simulink model "Diesel_Generator_Harness"  (R2025b)
settings: Solver=VariableStepAuto  StartTime=0.0  StopTime=15  RelTol=1e-3
PreLoadFcn:
  | GeneratorHarnessParam;
undefined symbols (not defined in the file): DiscIntNeverNeededParam, generator, machine, Ts
libraries: nesl_utility x16, ee_lib x14, fl_lib x7, eeGeneralControl x4, eeSmDC2C x1
settings Model: SimulationMode=accelerator  Creator=skota  LastModifiedBy=skota

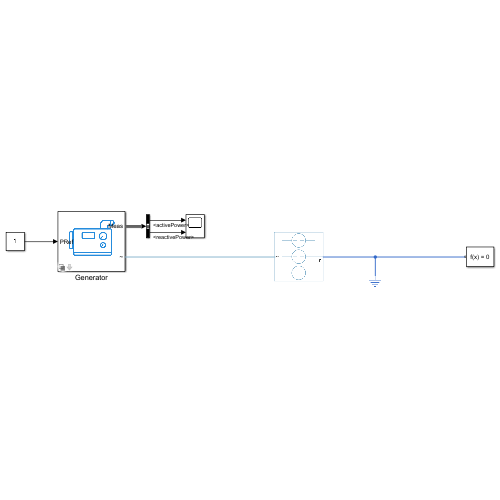
[thumbnail: Simulink's stored preview of the top-level diagram]
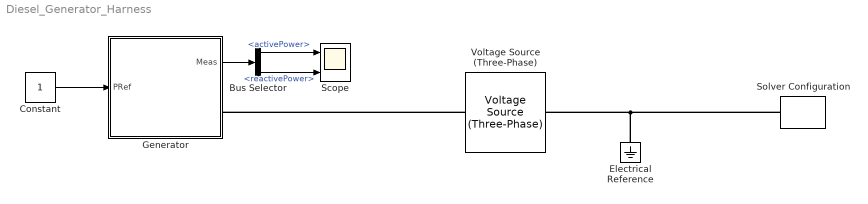
== system Diesel_Generator_Harness ==
  Bus Selector : BusSelector  OutputSignals=activePower,reactivePower
  Constant : Constant
  Electrical Reference : fl_lib/Electrical/Electrical Elements/Electrical Reference
  Generator : Subsystem  Variant=on  VariantControlMode=label  LabelModeActiveChoice=Detailed  mask(Generator){fidelity=Detailed, genRating=generator.rating, Vac=generator.Vac, frequency=generator.frequency, polePairs=generator.polePairs, pu_speed_reference=machine.speedReference, droop_percentage=machine.droop, pu_load_reference_setpoint=machine.loadReference, T_G=machine.timeConstandGovernor, T_CH=machine.timeConstantPrimeMover, base_torque=machine.baseTorque, pu_torque0=machine.initialTorque}
      mask prompts: fidelity "Modeling Option"; genRating "Generator Rating (kW)"; Vac "Rated AC side voltage (phase-phase RMS) (V)"; frequency "Rated electrical frequency at AC side (Hz)"; polePairs "Number of pole pairs"; pu_speed_reference "Speed reference, (pu)"; droop_percentage "Percentage droop, (%)"; pu_load_reference_setpoint "Load reference setpoint, (pu)"; T_G "Time constant of governor, (s)"; T_CH "Time constant of main inlet volumes and steam chest, (s)"; base_torque "Base torque, (N*m)"; pu_torque0 "Initial torque, (pu)"
      mask help:
      | This block models a Generator. The detailed variant models AVR, Exciter, Prime mover, and Governer. The simplified variant is based on load torque and a constant field circuit current. Select simplified mode for faster simulation using fixed efficiency and rated power.
      |
      | Provide load reference as input
      settings: CopyFcn=set_param(gcbh,'LinkStatus','none');
      mask Help: web('Generator.html')
      mask TypeOptions fidelity: Detailed | Simplified
      mask Callback fidelity:
      | detailedTabs = {'generatorDetailed','exciterParam','governerParam',};
      |     simplifiedTabs = {'generatorSimplified'};
      |     component.mask.fidelitySelection(detailedTabs,simplifiedTabs);
      |     component.mask.fidelitySelection;
      mask TypeOptions pu_speed_reference:
      | Detailed/Governor and
      | Prime Mover
      | /pu_speed_reference
      mask TypeOptions droop_percentage:
      | Detailed/Governor and
      | Prime Mover
      | /droop_percentage
      mask TypeOptions pu_load_reference_setpoint:
      | Detailed/Governor and
      | Prime Mover
      | /pu_load_reference_setpoint
      mask TypeOptions T_G:
      | Detailed/Governor and
      | Prime Mover
      | /T_G
      mask TypeOptions T_CH:
      | Detailed/Governor and
      | Prime Mover
      | /T_CH
      mask TypeOptions base_torque:
      | Detailed/Governor and
      | Prime Mover
      | /base_torque
      mask TypeOptions pu_torque0:
      | Detailed/Governor and
      | Prime Mover
      | /pu_torque0
      mask DialogControl generalDetailed Prompt: General
      mask DialogControl editMachine Prompt: Edit machine parameters
      mask DialogControl editMachine Callback:
      | blockFidelity = get_param(gcb,'fidelity');
      |     blockPath = [gcb,'/',blockFidelity,'/','Machine'];
      |     component.mask.openBlock(blockPath);
      mask DialogControl editInertia Prompt: Edit inertia parameters
      mask DialogControl editInertia Callback:
      | blockPath = [gcb,'/','Detailed','/','Inertia'];
      |     component.mask.openBlock(blockPath);
      mask DialogControl exciterParam Prompt: Exciter
      mask DialogControl fieldParam Prompt: Edit field circuit parameters
      mask DialogControl fieldParam Callback:
      | blockPath = [gcb,'/','Detailed','/','AVR and Exciter','/','Exciter'];
      |     component.mask.openBlock(blockPath);
      mask DialogControl avrParam Prompt: Edit AVR parameters
      mask DialogControl avrParam Callback:
      | blockPath = [gcb,'/','Detailed','/','AVR and Exciter','/','AVR'];
      |     component.mask.openBlock(blockPath);
      mask DialogControl governerParam Prompt: Governer and Prime Mover
  Scope : Scope  NumInputPorts=2
      settings: ActiveDisplayYMinimum=-1.6422066833599676  ActiveDisplayYMaximum=1.1874659177964262
  Solver Configuration : nesl_utility/Solver Configuration  PhysicalDomain=network_engine_domain  SubClassName=solver  LeftPortType=input  RightPortType=generic  Tones=[]  Harmonics=[]  SimulateNoise=off  Profile=off  UseLocalSampling=off  EnableSwitchedLinearOptims=on  FrequencyDomain=off  UseCCode=off  RelTol=0.001  AbsTol=0.001  MinStep=1e-09  ToWorkspace=off  RevertToSquareIcSolve=off  NumHomotopyIterations=100  PhasorMode=off  PhasorModeNumHarmonics=1  ConsistencySolver=NEWTON_XTOL_AFTER_FTOL  IndexReductionMethod=DerivativeReplacement  DoDC=off  ResidualTolerance=1e-09  ConsistencyTolSource=GLOBAL  ConsistencyAbsTol=0.001  ConsistencyRelTol=0.001  ConsistencyTolFactor=0.001  UseLocalSolver=on  LocalSolverChoice=NE_BACKWARD_EULER_ADVANCER  ResolveIndetEquations=on  FunctionEvalNumThread=1  LocalSolverSampleTime=5e-5  DoFixedCost=off  MaxNonlinIter=3  MaxModeIter=2  ComputeImpulses=off  ImpulseIterations=2  LinearAlgebra=auto  LinearAlgebraNumThread=0  EquationFormulation=NE_TIME_EF  DelaysMemoryBudget=1024  AutomaticFiltering=on  FilteringTimeConstant=0.001  PartitionStorageMethod=AS_NEEDED  PartitionMemoryBudget=1024  PartitionMethod=ROBUST  MultibodyUseLocalSolver=off  MultibodyLocalSolverChoice=ODE1  MultibodyLocalSolverSampleTime=0.001
  Voltage Source (Three-Phase) : ee_lib/Sources/Voltage Source (Three-Phase)  vline_rms=480 V  shift=0 deg  freq=60 Hz  impedance_option=1  SShortCircuit=100e6 A*V  XR=20  R=0.01 Ohm  L=3.97e-4 H  harmonic_option=0  harmonic_orders=[5, 7, 11, 13]  harmonic_ratios=[.1, .1, .1, .1]  G_parasitic=0 1/Ohm  I_specify=off  I_priority=None  I=[0, 0, 0] A  I_nominal_specify=off  I_nominal_value=1  I_nominal_unit=A
  wires:
  Bus Selector/1 -> Scope/1  "<activePower>"
  Bus Selector/2 -> Scope/2  "<reactivePower>"
  Constant/1 -> Generator/1(PRef)
  Generator/1(Meas) -> Bus Selector/1
  connections:
  Electrical Reference/LConn1 -- Solver Configuration/RConn1 -- Voltage Source (Three-Phase)/LConn1
  Voltage Source (Three-Phase)/RConn1 -- Generator/RConn1

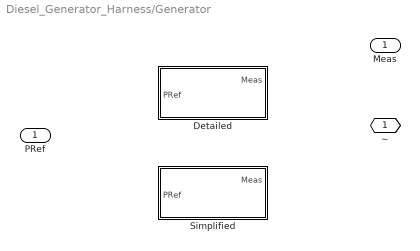
== system Diesel_Generator_Harness/Generator ==
  PRef : Inport
  Detailed : Subsystem  VariantControl=Detailed
  Simplified : Subsystem  VariantControl=Simplified
  ~ : PMIOPort  Side=Right
  Meas : Outport

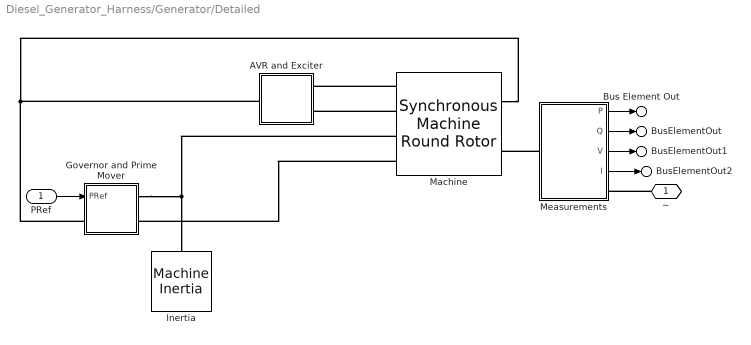
== system Diesel_Generator_Harness/Generator/Detailed ==
  PRef : Inport
  AVR and Exciter : Subsystem
  "Governor and Prime Mover " : Subsystem  mask(Governor and Prime Mover){pu_speed_reference=pu_speed_reference, droop_percentage=droop_percentage, pu_load_reference_setpoint=pu_load_reference_setpoint, T_G=T_G, T_CH=T_CH, base_torque=base_torque, pu_torque0=pu_torque0}
      mask prompts: pu_speed_reference "Speed reference, (pu)"; droop_percentage "Percentage droop, (%)"; pu_load_reference_setpoint "Load reference setpoint, (pu)"; T_G "Time constant of governor, (s)"; T_CH "Time constant of main inlet volumes and steam chest, (s)"; base_torque "Base torque, (N*m)"; pu_torque0 "Initial torque, (pu)"
      mask help:
      | Implements a synchronous machine governor and prime mover. The prime mover is a non-reheat steam turbine.
      |
      | The input to the block is a per-unit synchronous machine measurement vector.
      |
      | R and C are mechanical rotational ports.
  Inertia : ee_lib/Electromechanical/Mechanical/Machine Inertia  SRated=genRating*1000 V*A  FRated=frequency Hz  nPolePairs=polePairs  inertia_option=2  J=0.5754*200 kg*m^2  H=3.525*2 s*W/V/A  damper_option=2  D=39.0509 N*m/(rad/s)  pu_D=0.01  initialization_option=2  fMechanical0=60 Hz  fElectrical0=frequency Hz
      settings: InternalSimscapePortConfiguration="{\"Bottom\":[],\"Left\":[{\"id\":\"R\",\"label\":\"R\",\"type\":\"foundation.mechanical.rotational.rotational\"}],\"Right\":[],\"Top\":[]}"
  Machine : ee_lib/Electromechanical/Synchronous/Synchronous Machine Round Rotor  port_option=ee.enum.threePhasePort.composite  SRated=genRating*1000 A*V  VRated=Vac V  FRated=frequency Hz  nPolePairs=polePairs  param_option=ee.enum.sm.parameterization.standard  fieldCircuitParameterization_option=ee.enum.sm.fieldparameterization.current  baseEfd=92.95 V  baseIfd=machine.fieldCurrent A  zero_sequence=ee.enum.park.zerosequence.exclude  axes_param=ee.enum.rotorangle.daxis  Ladu=1.66  Laqu=1.61  L0=0.15  Ll=0.05  Ra=machine.Ra/2  Lfd=0.165  Rfd=0.0006  L1d=0.1713  R1d=0.0284  L1q=0.7252  R1q=0.00619  L2q=0.125  R2q=0.02368  Xl=machine.Xl  Xd=machine.Xd  Xq=machine.Xq  X0=0.06  Xdd=machine.XdTransient  Xqd=machine.XqTransient  Xddd=machine.XdSubTransient  Xqdd=machine.XqSubTransient  d_option=ee.enum.circuit.open  Td0d=machine.tauDAxisTransient s  Tdd=0.03 s  Td0dd=machine.tauDAxisSubTransient s  Tddd=0.008 s  q_option=ee.enum.circuit.open  Tq0d=machine.tauQAxisTransient s  Tqd=0.03 s  Tq0dd=machine.tauQAxisSubTransient s  Tqdd=0.008 s  saturation_option=ee.enum.saturation.exclude  saturation_ifd=[0, .48, .76, 1.38, 1.79]  saturation_Vag=[0, .8, 1.08, 1.31, 1.4]  initialization_option=ee.enum.sm.initialization.steadystate  source_type=ee.enum.sm.load_flow_source_type.Swing  Vmag0=machine.voltage V  Vang0=0 deg  Pt0=0 A*V  Qt0=0 A*V  minimum_pu=0.95  phase_search_range=[-inf, inf] deg  gmin=1e-6 S  connection_option=ee.enum.Connection.wye  num_q_dampers=2  rotor_offset=-pi / 2 rad  pu_psid_specify=off  pu_psid_priority=None  pu_psid=0  pu_psid_nominal_specify=off  pu_psid_nominal_value=1  pu_psid_nominal_unit=1  pu_psiq_specify=off  pu_psiq_priority=None  pu_psiq=0  pu_psiq_nominal_specify=off  pu_psiq_nominal_value=1  pu_psiq_nominal_unit=1  pu_psifd_specify=off  pu_psifd_priority=None  pu_psifd=0  pu_psifd_nominal_specify=off  pu_psifd_nominal_value=1  pu_psifd_nominal_unit=1  pu_psi1d_specify=off  pu_psi1d_priority=None  pu_psi1d=0  pu_psi1d_nominal_specify=off  pu_psi1d_nominal_value=1  pu_psi1d_nominal_unit=1  pu_psi1q_specify=off  pu_psi1q_priority=None  pu_psi1q=0  pu_psi1q_nominal_specify=off  pu_psi1q_nominal_value=1  pu_psi1q_nominal_unit=1  pu_psi2q_specify=off  pu_psi2q_priority=None  pu_psi2q=0  pu_psi2q_nominal_specify=off  pu_psi2q_nominal_value=1  pu_psi2q_nominal_unit=1  angular_position_diff_specify=off  angular_position_diff_priority=None  angular_position_diff=180 deg  angular_position_diff_nominal_specify=off  angular_position_diff_nominal_value=1  angular_position_diff_nominal_unit=deg  Tmeas=298.15 K  alpha=3.93e-3 1/K  stator_thermal_mass=100 J/K  rotor_thermal_mass=200 J/K  temperatureA_specify=off  temperatureA_priority=High  temperatureA=25 degC  temperatureA_nominal_specify=off  temperatureA_nominal_value=1  temperatureA_nominal_unit=degC  temperatureB_specify=off  temperatureB_priority=High  temperatureB=25 degC  temperatureB_nominal_specify=off  temperatureB_nominal_value=1  temperatureB_nominal_unit=degC  temperatureC_specify=off  temperatureC_priority=High  temperatureC=25 degC  temperatureC_nominal_specify=off  temperatureC_nominal_value=1  temperatureC_nominal_unit=degC  temperatureR_specify=off  temperatureR_priority=High  temperatureR=25 degC  temperatureR_nominal_specify=off  temperatureR_nominal_value=1  temperatureR_nominal_unit=degC
      settings: InternalSimscapePortConfiguration="{\"Bottom\":[],\"Left\":[{\"id\":\"fd_p\",\"label\":\"fd+\",\"type\":\"foundation.electrical.electrical\"},{\"id\":\"fd_n\",\"label\":\"fd-\",\"type\":\"foundation.electrical.electrical\"},{\"id\":\"R\",\"label\":\"R\",\"type\":\"foundation.mechanical.rotational.rotational\"},{\"id\":\"C\",\"label\":\"C\",\"type\":\"foundation.mechanical.rotational.rotational\"}],\"Right\":[{\"id\":\"pu_output\",\"label\":\"pu\",\"type\":\"output\"},{\"id\":\"N\",\"label\":\"~\",\"type\":\"foundation.electrical.three_phase\"}],\"Top\":[]}"
  Measurements : Subsystem
  ~ : PMIOPort  Side=Right
  Bus Element Out : Outport  PortName=Meas  Element=activePower
  BusElementOut : Outport  PortName=Meas  Element=reactivePower
  BusElementOut1 : Outport  PortName=Meas  Element=voltage
  BusElementOut2 : Outport  PortName=Meas  Element=current
  wires:
  Measurements/4(I) -> BusElementOut2/1
  Measurements/3(V) -> BusElementOut1/1
  Measurements/1(P) -> Bus Element Out/1
  Measurements/2(Q) -> BusElementOut/1
  PRef/1 -> "Governor and Prime Mover "/1(PRef)
  connections:
  ~/RConn1 -- Measurements/RConn1
  Measurements/LConn1 -- Machine/RConn2
  Machine/LConn1 -- AVR and Exciter/RConn1
  Machine/LConn4 -- "Governor and Prime Mover "/RConn2
  "Governor and Prime Mover "/RConn1 -- Machine/LConn3 -- Inertia/LConn1
  "Governor and Prime Mover "/LConn1 -- Machine/RConn1 -- AVR and Exciter/LConn1
  Machine/LConn2 -- AVR and Exciter/RConn2

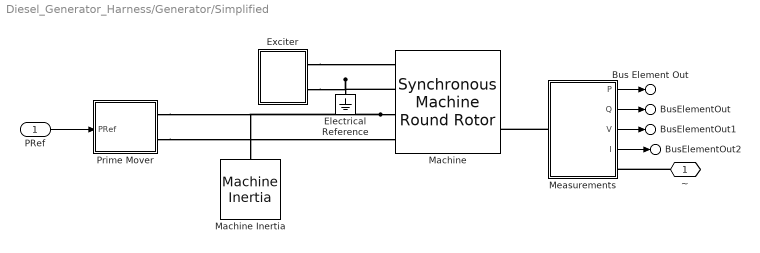
== system Diesel_Generator_Harness/Generator/Simplified ==
  PRef : Inport
  Electrical Reference : fl_lib/Electrical/Electrical Elements/Electrical Reference
  Exciter : Subsystem
  Machine : ee_lib/Electromechanical/Synchronous/Synchronous Machine Round Rotor  port_option=ee.enum.threePhasePort.composite  SRated=genRating kW  VRated=Vac V  FRated=frequency Hz  nPolePairs=polePairs  param_option=ee.enum.sm.parameterization.standard  fieldCircuitParameterization_option=ee.enum.sm.fieldparameterization.voltage  baseEfd=100 V  baseIfd=1300 A  zero_sequence=ee.enum.park.zerosequence.exclude  axes_param=ee.enum.rotorangle.daxis  Ladu=1.66  Laqu=1.61  L0=0.15  Ll=0.05  Ra=0.03/5  Lfd=0.165  Rfd=0.0006  L1d=0.1713  R1d=0.0284  L1q=0.7252  R1q=0.00619  L2q=0.125  R2q=0.02368  Xl=0.05/5  Xd=1.72/5  Xq=0.79/5  X0=0.06  Xdd=0.13/5  Xqd=0.17/3  Xddd=0.09/5  Xqdd=0.12/5  d_option=ee.enum.circuit.short  Td0d=0.75 s  Tdd=0.03 s  Td0dd=0.03 s  Tddd=0.008 s  q_option=ee.enum.circuit.open  Tq0d=0.6 s  Tqd=0.03 s  Tq0dd=0.02 s  Tqdd=0.008 s  saturation_option=ee.enum.saturation.exclude  saturation_ifd=[0, .48, .76, 1.38, 1.79]  saturation_Vag=[0, .8, 1.08, 1.31, 1.4]  initialization_option=ee.enum.sm.initialization.steadystate  source_type=ee.enum.sm.load_flow_source_type.Swing  Vmag0=6600 V  Vang0=0 deg  Pt0=0 A*V  Qt0=0 A*V  minimum_pu=0.95  phase_search_range=[-inf, inf] deg  gmin=1e-4 S  connection_option=ee.enum.Connection.wye  num_q_dampers=2  rotor_offset=-pi / 2 rad  pu_psid_specify=off  pu_psid_priority=None  pu_psid=0  pu_psid_nominal_specify=off  pu_psid_nominal_value=1  pu_psid_nominal_unit=1  pu_psiq_specify=off  pu_psiq_priority=None  pu_psiq=0  pu_psiq_nominal_specify=off  pu_psiq_nominal_value=1  pu_psiq_nominal_unit=1  pu_psifd_specify=off  pu_psifd_priority=None  pu_psifd=0  pu_psifd_nominal_specify=off  pu_psifd_nominal_value=1  pu_psifd_nominal_unit=1  pu_psi1d_specify=off  pu_psi1d_priority=None  pu_psi1d=0  pu_psi1d_nominal_specify=off  pu_psi1d_nominal_value=1  pu_psi1d_nominal_unit=1  pu_psi1q_specify=off  pu_psi1q_priority=None  pu_psi1q=0  pu_psi1q_nominal_specify=off  pu_psi1q_nominal_value=1  pu_psi1q_nominal_unit=1  pu_psi2q_specify=off  pu_psi2q_priority=None  pu_psi2q=0  pu_psi2q_nominal_specify=off  pu_psi2q_nominal_value=1  pu_psi2q_nominal_unit=1  angular_position_diff_specify=off  angular_position_diff_priority=None  angular_position_diff=180 deg  angular_position_diff_nominal_specify=off  angular_position_diff_nominal_value=1  angular_position_diff_nominal_unit=deg  Tmeas=298.15 K  alpha=3.93e-3 1/K  stator_thermal_mass=100 J/K  rotor_thermal_mass=200 J/K  temperatureA_specify=off  temperatureA_priority=High  temperatureA=25 degC  temperatureA_nominal_specify=off  temperatureA_nominal_value=1  temperatureA_nominal_unit=degC  temperatureB_specify=off  temperatureB_priority=High  temperatureB=25 degC  temperatureB_nominal_specify=off  temperatureB_nominal_value=1  temperatureB_nominal_unit=degC  temperatureC_specify=off  temperatureC_priority=High  temperatureC=25 degC  temperatureC_nominal_specify=off  temperatureC_nominal_value=1  temperatureC_nominal_unit=degC  temperatureR_specify=off  temperatureR_priority=High  temperatureR=25 degC  temperatureR_nominal_specify=off  temperatureR_nominal_value=1  temperatureR_nominal_unit=degC
      settings: InternalSimscapePortConfiguration="{\"Bottom\":[],\"Left\":[{\"id\":\"fd_p\",\"label\":\"fd+\",\"type\":\"foundation.electrical.electrical\"},{\"id\":\"fd_n\",\"label\":\"fd-\",\"type\":\"foundation.electrical.electrical\"},{\"id\":\"R\",\"label\":\"R\",\"type\":\"foundation.mechanical.rotational.rotational\"},{\"id\":\"C\",\"label\":\"C\",\"type\":\"foundation.mechanical.rotational.rotational\"}],\"Right\":[{\"id\":\"pu_output\",\"label\":\"pu\",\"type\":\"output\"},{\"id\":\"N\",\"label\":\"~\",\"type\":\"foundation.electrical.three_phase\"}],\"Top\":[]}"
  Machine Inertia : ee_lib/Electromechanical/Mechanical/Machine Inertia  SRated=genRating*1000 V*A  FRated=frequency Hz  nPolePairs=polePairs  inertia_option=1  J=0.5754 kg*m^2  H=3.525 s*W/V/A  damper_option=2  D=39.0509 N*m/(rad/s)  pu_D=0.01  initialization_option=2  fMechanical0=60 Hz  fElectrical0=60 Hz
      settings: InternalSimscapePortConfiguration="{\"Bottom\":[],\"Left\":[{\"id\":\"R\",\"label\":\"R\",\"type\":\"foundation.mechanical.rotational.rotational\"}],\"Right\":[],\"Top\":[]}"
  Measurements : Subsystem
  Prime Mover : Subsystem
  ~ : PMIOPort  Side=Right
  Bus Element Out : Outport  PortName=Meas  Element=activePower
  BusElementOut : Outport  PortName=Meas  Element=reactivePower
  BusElementOut1 : Outport  PortName=Meas  Element=voltage
  BusElementOut2 : Outport  PortName=Meas  Element=current
  wires:
  Measurements/2(Q) -> BusElementOut/1
  Measurements/1(P) -> Bus Element Out/1
  Measurements/3(V) -> BusElementOut1/1
  Measurements/4(I) -> BusElementOut2/1
  PRef/1 -> Prime Mover/1(PRef)
  connections:
  Measurements/LConn1 -- Machine/RConn2
  ~/RConn1 -- Measurements/RConn1
  Prime Mover/RConn2 -- Machine/LConn4
  Exciter/RConn1 -- Machine/LConn1
  Machine/LConn3 -- Prime Mover/RConn1 -- Machine Inertia/LConn1
  Electrical Reference/LConn1 -- Machine/LConn2 -- Exciter/RConn2

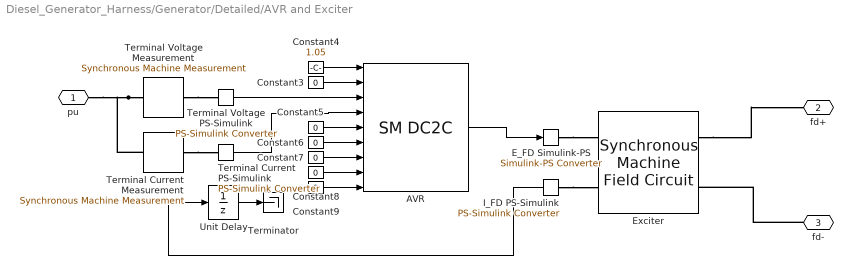
== system Diesel_Generator_Harness/Generator/Detailed/AVR and Exciter ==
  AVR : eeSmDC2C/SM DC2C  E_FD0=1.01  Ts=Ts  R_C=0  X_C=0  T_R=0  K_A=300  T_A=0.06  T_B=0  T_C=0  K_F=0.058  T_F=0.62  V_Rmax=4.5  V_Rmin=-4.5  oelInputLocation=Unused  uelInputLocation=Unused  sclInputLocation=Unused  K_E=1  T_E=1.33  E_FDmin=-99  E_1=3.05  S_E_E1=0.279  E_2=2.29  S_E_E2=0.117
  Constant{3,5..9} (6 alike) : Constant  Value=0
  Constant4 : Constant  Value=1.05
  "E_FD Simulink-PS " : nesl_utility/Simulink-PS Converter  PhysicalDomain=network_engine_domain  SubClassName=ps_input  LeftPortType=input  RightPortType=output  PseudoPeriodic=off  Frequencies=[]  NoiseDistribution=none  NoiseParameters=[]  Unit=1  AffineConversion=off  FilteringAndDerivatives=provide  SimscapeFilterOrder=1  InputFilterTimeConstant=.001  UdotUserProvided=0
  Exciter : ee_lib/Electromechanical/Synchronous/Synchronous Machine Field Circuit  unit_option=ee.enum.unit.pu  SRated=machine.ratedPower V*A  FRated=machine.frequency Hz  fieldCircuitParameterization_option=ee.enum.sm.fieldparameterization.current  baseEfd=200 V  baseIfd=machine.fieldCurrent A  parameterization_option=2  Ladu=1.66  Rfd=0.0006  Xl=machine.Xl  Xd=machine.Xd  Xdd=machine.XdTransient  Xddd=machine.XdSubTransient  d_option=ee.enum.circuit.open  Td0d=machine.tauDAxisTransient s  Tdd=0.03 s  Td0dd=machine.tauDAxisSubTransient s  Tddd=0.008 s
      settings: InternalSimscapePortConfiguration="{\"Bottom\":[],\"Left\":[{\"id\":\"Efd_pu\",\"label\":\"Efd_pu\",\"type\":\"input\"},{\"id\":\"Ifd_pu\",\"label\":\"Ifd_pu\",\"type\":\"output\"}],\"Right\":[{\"id\":\"fd_p\",\"label\":\"fd+\",\"type\":\"foundation.electrical.electrical\"},{\"id\":\"fd_n\",\"label\":\"fd-\",\"type\":\"foundation.electrical.electrical\"}],\"Top\":[]}"
  I_FD PS-Simulink : nesl_utility/PS-Simulink Converter  PhysicalDomain=network_engine_domain  SubClassName=ps_output  LeftPortType=input  RightPortType=output  PseudoPeriodic=off  Frequencies=[]  VectorFormat=1-D array  Unit=1  AffineConversion=off
  Terminal Current Measurement : ee_lib/Electromechanical/Synchronous/Synchronous Machine Measurement  output_idx=15
      settings: InternalSimscapePortConfiguration="{\"Bottom\":[],\"Left\":[{\"id\":\"pu_input\",\"label\":\"pu\",\"type\":\"input\"}],\"Right\":[{\"id\":\"pu_output\",\"label\":\"o\",\"type\":\"output\"}],\"Top\":[]}"
  Terminal Current PS-Simulink : nesl_utility/PS-Simulink Converter  PhysicalDomain=network_engine_domain  SubClassName=ps_output  LeftPortType=input  RightPortType=output  PseudoPeriodic=off  Frequencies=[]  VectorFormat=1-D array  Unit=1  AffineConversion=off
  Terminal Voltage Measurement : ee_lib/Electromechanical/Synchronous/Synchronous Machine Measurement  output_idx=14
      settings: InternalSimscapePortConfiguration="{\"Bottom\":[],\"Left\":[{\"id\":\"pu_input\",\"label\":\"pu\",\"type\":\"input\"}],\"Right\":[{\"id\":\"pu_output\",\"label\":\"o\",\"type\":\"output\"}],\"Top\":[]}"
  Terminal Voltage PS-Simulink : nesl_utility/PS-Simulink Converter  PhysicalDomain=network_engine_domain  SubClassName=ps_output  LeftPortType=input  RightPortType=output  PseudoPeriodic=off  Frequencies=[]  VectorFormat=1-D array  Unit=1  AffineConversion=off
  Terminator : Terminator
  Unit Delay : UnitDelay  InitialCondition=1.32943  SampleTime=-1
  pu : PMIOPort  Side=Left
  fd+ : PMIOPort  Port=2  Side=Right
  fd- : PMIOPort  Port=3  Side=Right
  wires:
  Unit Delay/1 -> Terminator/1
  I_FD PS-Simulink/1 -> Unit Delay/1
  Terminal Voltage PS-Simulink/1 -> AVR/3
  Constant3/1 -> AVR/2
  Constant4/1 -> AVR/1
  Constant5/1 -> AVR/5
  Constant6/1 -> AVR/6
  Constant7/1 -> AVR/7
  Constant8/1 -> AVR/8
  Constant9/1 -> AVR/9
  AVR/1 -> "E_FD Simulink-PS "/1
  Terminal Current PS-Simulink/1 -> AVR/4
  connections:
  "E_FD Simulink-PS "/RConn1 -- Exciter/LConn1
  I_FD PS-Simulink/LConn1 -- Exciter/LConn2
  fd-/RConn1 -- Exciter/RConn2
  Exciter/RConn1 -- fd+/RConn1
  Terminal Voltage Measurement/LConn1 -- Terminal Current Measurement/LConn1 -- pu/RConn1
  Terminal Voltage Measurement/RConn1 -- Terminal Voltage PS-Simulink/LConn1
  Terminal Current Measurement/RConn1 -- Terminal Current PS-Simulink/LConn1

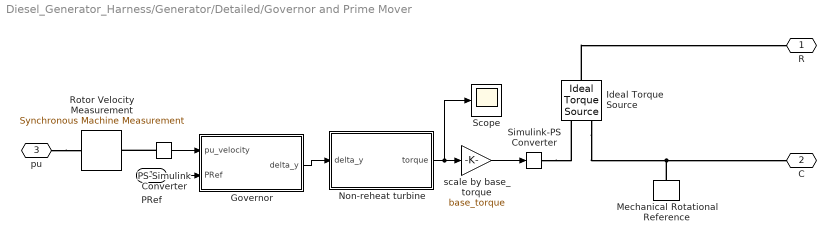
== system Diesel_Generator_Harness/Generator/Detailed/Governor and Prime Mover  ==
  PRef : Inport
  Governor : Subsystem
  Ideal Torque Source : fl_lib/Mechanical/Mechanical Sources/Ideal Torque Source
  Mechanical Rotational Reference : fl_lib/Mechanical/Rotational Elements/Mechanical Rotational Reference
  Non-reheat turbine : Subsystem
  PS-Simulink Converter : nesl_utility/PS-Simulink Converter  PhysicalDomain=network_engine_domain  SubClassName=ps_output  LeftPortType=input  RightPortType=output  PseudoPeriodic=off  Frequencies=[]  VectorFormat=1-D array  Unit=1  AffineConversion=off
  Rotor Velocity Measurement : ee_lib/Electromechanical/Synchronous/Synchronous Machine Measurement  output_idx=4
      settings: InternalSimscapePortConfiguration="{\"Bottom\":[],\"Left\":[{\"id\":\"pu_input\",\"label\":\"pu\",\"type\":\"input\"}],\"Right\":[{\"id\":\"pu_output\",\"label\":\"o\",\"type\":\"output\"}],\"Top\":[]}"
  Scope : Scope
  Simulink-PS Converter : nesl_utility/Simulink-PS Converter  PhysicalDomain=network_engine_domain  SubClassName=ps_input  LeftPortType=input  RightPortType=output  PseudoPeriodic=off  Frequencies=[]  NoiseDistribution=none  NoiseParameters=[]  Unit=1  AffineConversion=off  FilteringAndDerivatives=zero  SimscapeFilterOrder=1  InputFilterTimeConstant=0.001  UdotUserProvided=1
  scale by base_torque : Gain  Gain=base_torque
  R : PMIOPort  Side=Right
  C : PMIOPort  Port=2  Side=Right
  pu : PMIOPort  Port=3  Side=Left
  wires:
  PRef/1 -> Governor/2(PRef)
  scale by base_torque/1 -> Simulink-PS Converter/1
  Non-reheat turbine/1(torque) -> scale by base_torque/1, Scope/1
  Governor/1(delta_y) -> Non-reheat turbine/1(delta_y)
  PS-Simulink Converter/1 -> Governor/1(pu_velocity)
  connections:
  Simulink-PS Converter/RConn1 -- Ideal Torque Source/RConn1
  PS-Simulink Converter/LConn1 -- Rotor Velocity Measurement/RConn1
  pu/RConn1 -- Rotor Velocity Measurement/LConn1
  Ideal Torque Source/LConn1 -- R/RConn1
  Mechanical Rotational Reference/LConn1 -- Ideal Torque Source/RConn2 -- C/RConn1

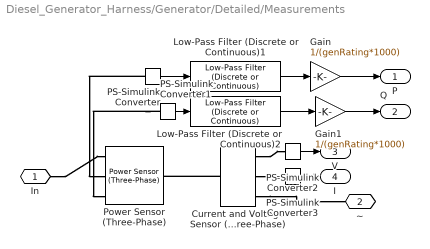
== system Diesel_Generator_Harness/Generator/Detailed/Measurements ==
  Current and Voltage Sensor (Three-Phase) : ee_lib/Sensors & Transducers/Current and Voltage Sensor (Three-Phase)  vMeasurementType=ee.enum.vmeasurement.ll  outputUnit=ee.enum.unit.pu  SRated=genRating*1000 A*V  VRated=Vac V  I_specify=off  I_priority=None  I=[0, 0, 0] A  I_nominal_specify=off  I_nominal_value=1  I_nominal_unit=A  V_specify=off  V_priority=None  V=[0, 0, 0] V  V_nominal_specify=off  V_nominal_value=1  V_nominal_unit=V
      settings: InternalSimscapePortConfiguration="{\"Bottom\":[],\"Left\":[{\"id\":\"N1\",\"label\":\"~1\",\"type\":\"foundation.electrical.three_phase\"}],\"Right\":[{\"id\":\"V_output\",\"label\":\"V\",\"type\":\"output\"},{\"id\":\"I_output\",\"label\":\"I\",\"type\":\"output\"},{\"id\":\"N2\",\"label\":\"~2\",\"type\":\"foundation.electrical.three_phase\"}],\"Top\":[]}"
  Gain : Gain  Gain=1/(genRating*1000)
  Gain1 : Gain  Gain=1/(genRating*1000)
  Low-Pass Filter (Discrete or Continuous)1 : eeGeneralControl/Low-Pass Filter (Discrete or Continuous)  K=1  T=0.1  B=inf  A=-inf  init_option=Inherited from block input  x0=0  Ts=-1
  Low-Pass Filter (Discrete or Continuous)2 : eeGeneralControl/Low-Pass Filter (Discrete or Continuous)  K=1  T=0.1  B=inf  A=-inf  init_option=Inherited from block input  x0=0  Ts=-1
  PS-Simulink Converter{,1..3} (4 alike) : nesl_utility/PS-Simulink Converter  PhysicalDomain=network_engine_domain  SubClassName=ps_output  LeftPortType=input  RightPortType=output  PseudoPeriodic=off  Frequencies=[]  VectorFormat=inherit  Unit=inherit  AffineConversion=off
  Power Sensor (Three-Phase) : ee_lib/Sensors & Transducers/Power Sensor (Three-Phase)  load_type=ee.enum.passive.type_balanced.balanced  f0=60 Hz
      settings: InternalSimscapePortConfiguration="{\"Bottom\":[],\"Left\":[{\"id\":\"N1\",\"label\":\"~1\",\"type\":\"foundation.electrical.three_phase\"}],\"Right\":[{\"id\":\"N2\",\"label\":\"~2\",\"type\":\"foundation.electrical.three_phase\"}],\"Top\":[{\"id\":\"Pm\",\"label\":\"P\",\"type\":\"output\"},{\"id\":\"Qm\",\"label\":\"Q\",\"type\":\"output\"}]}"
  In : PMIOPort  Side=Left
  ~ : PMIOPort  Port=2  Side=Right
  P : Outport
  Q : Outport  Port=2
  V : Outport  Port=3
  I : Outport  Port=4
  wires:
  Gain1/1 -> Q/1
  Gain/1 -> P/1
  PS-Simulink Converter3/1 -> I/1
  PS-Simulink Converter2/1 -> V/1
  Low-Pass Filter (Discrete or Continuous)2/1 -> Gain1/1
  Low-Pass Filter (Discrete or Continuous)1/1 -> Gain/1
  PS-Simulink Converter1/1 -> Low-Pass Filter (Discrete or Continuous)2/1
  PS-Simulink Converter/1 -> Low-Pass Filter (Discrete or Continuous)1/1
  connections:
  Current and Voltage Sensor (Three-Phase)/RConn2 -- PS-Simulink Converter3/LConn1
  Current and Voltage Sensor (Three-Phase)/LConn1 -- Power Sensor (Three-Phase)/RConn1
  PS-Simulink Converter1/LConn1 -- Power Sensor (Three-Phase)/LConn3
  Current and Voltage Sensor (Three-Phase)/RConn3 -- ~/RConn1
  In/RConn1 -- Power Sensor (Three-Phase)/LConn1
  PS-Simulink Converter/LConn1 -- Power Sensor (Three-Phase)/LConn2
  Current and Voltage Sensor (Three-Phase)/RConn1 -- PS-Simulink Converter2/LConn1

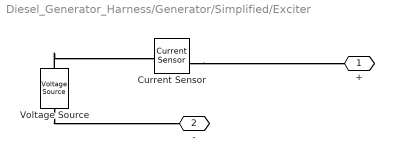
== system Diesel_Generator_Harness/Generator/Simplified/Exciter ==
  Current Sensor : fl_lib/Electrical/Electrical Sensors/Current Sensor
  Voltage Source : ee_lib/Sources/Voltage Source  dc_voltage=120 V  ac_voltage=0 V  ac_shift=0 rad  ac_frequency=frequency Hz  noise_mode=ee.enum.sources.noise.Disabled  PSD=0 V^2/Hz  sample_time=1e-3 s  repeatability=ee.enum.sources.repeatability.NotRepeatable  user_seed=0  auto_seed=3890346746  i_specify=off  i_priority=None  i=0 A  i_nominal_specify=off  i_nominal_value=1  i_nominal_unit=A  v_specify=off  v_priority=None  v=0 V  v_nominal_specify=off  v_nominal_value=1  v_nominal_unit=V
  + : PMIOPort  Side=Right
  - : PMIOPort  Port=2  Side=Right
  connections:
  Voltage Source/LConn1 -- Current Sensor/LConn1
  Current Sensor/RConn2 -- +/RConn1
  Voltage Source/RConn1 -- -/RConn1

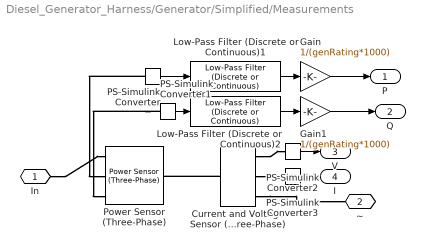
== system Diesel_Generator_Harness/Generator/Simplified/Measurements ==
  Current and Voltage Sensor (Three-Phase) : ee_lib/Sensors & Transducers/Current and Voltage Sensor (Three-Phase)  vMeasurementType=ee.enum.vmeasurement.ll  outputUnit=ee.enum.unit.pu  SRated=genRating*1000 A*V  VRated=Vac V  I_specify=off  I_priority=None  I=[0, 0, 0] A  I_nominal_specify=off  I_nominal_value=1  I_nominal_unit=A  V_specify=off  V_priority=None  V=[0, 0, 0] V  V_nominal_specify=off  V_nominal_value=1  V_nominal_unit=V
      settings: InternalSimscapePortConfiguration="{\"Bottom\":[],\"Left\":[{\"id\":\"N1\",\"label\":\"~1\",\"type\":\"foundation.electrical.three_phase\"}],\"Right\":[{\"id\":\"V_output\",\"label\":\"V\",\"type\":\"output\"},{\"id\":\"I_output\",\"label\":\"I\",\"type\":\"output\"},{\"id\":\"N2\",\"label\":\"~2\",\"type\":\"foundation.electrical.three_phase\"}],\"Top\":[]}"
  Gain : Gain  Gain=1/(genRating*1000)
  Gain1 : Gain  Gain=1/(genRating*1000)
  Low-Pass Filter (Discrete or Continuous)1 : eeGeneralControl/Low-Pass Filter (Discrete or Continuous)  K=1  T=0.1  B=inf  A=-inf  init_option=Inherited from block input  x0=0  Ts=-1
  Low-Pass Filter (Discrete or Continuous)2 : eeGeneralControl/Low-Pass Filter (Discrete or Continuous)  K=1  T=0.1  B=inf  A=-inf  init_option=Inherited from block input  x0=0  Ts=-1
  PS-Simulink Converter{,1..3} (4 alike) : nesl_utility/PS-Simulink Converter  PhysicalDomain=network_engine_domain  SubClassName=ps_output  LeftPortType=input  RightPortType=output  PseudoPeriodic=off  Frequencies=[]  VectorFormat=inherit  Unit=inherit  AffineConversion=off
  Power Sensor (Three-Phase) : ee_lib/Sensors & Transducers/Power Sensor (Three-Phase)  load_type=ee.enum.passive.type_balanced.balanced  f0=60 Hz
      settings: InternalSimscapePortConfiguration="{\"Bottom\":[],\"Left\":[{\"id\":\"N1\",\"label\":\"~1\",\"type\":\"foundation.electrical.three_phase\"}],\"Right\":[{\"id\":\"N2\",\"label\":\"~2\",\"type\":\"foundation.electrical.three_phase\"}],\"Top\":[{\"id\":\"Pm\",\"label\":\"P\",\"type\":\"output\"},{\"id\":\"Qm\",\"label\":\"Q\",\"type\":\"output\"}]}"
  In : PMIOPort  Side=Left
  ~ : PMIOPort  Port=2  Side=Right
  P : Outport
  Q : Outport  Port=2
  V : Outport  Port=3
  I : Outport  Port=4
  wires:
  Gain1/1 -> Q/1
  Gain/1 -> P/1
  PS-Simulink Converter3/1 -> I/1
  PS-Simulink Converter2/1 -> V/1
  Low-Pass Filter (Discrete or Continuous)2/1 -> Gain1/1
  Low-Pass Filter (Discrete or Continuous)1/1 -> Gain/1
  PS-Simulink Converter1/1 -> Low-Pass Filter (Discrete or Continuous)2/1
  PS-Simulink Converter/1 -> Low-Pass Filter (Discrete or Continuous)1/1
  connections:
  Current and Voltage Sensor (Three-Phase)/RConn2 -- PS-Simulink Converter3/LConn1
  Current and Voltage Sensor (Three-Phase)/LConn1 -- Power Sensor (Three-Phase)/RConn1
  PS-Simulink Converter1/LConn1 -- Power Sensor (Three-Phase)/LConn3
  Current and Voltage Sensor (Three-Phase)/RConn3 -- ~/RConn1
  In/RConn1 -- Power Sensor (Three-Phase)/LConn1
  PS-Simulink Converter/LConn1 -- Power Sensor (Three-Phase)/LConn2
  Current and Voltage Sensor (Three-Phase)/RConn1 -- PS-Simulink Converter2/LConn1

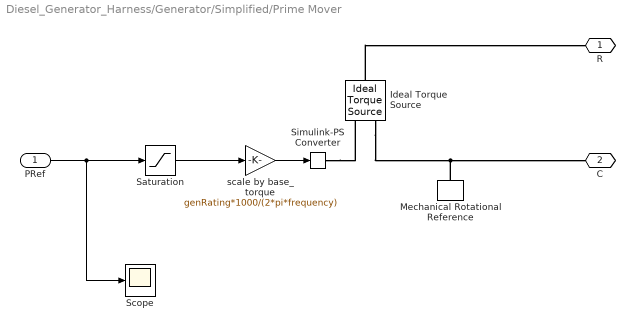
== system Diesel_Generator_Harness/Generator/Simplified/Prime Mover ==
  PRef : Inport
  Ideal Torque Source : fl_lib/Mechanical/Mechanical Sources/Ideal Torque Source
  Mechanical Rotational Reference : fl_lib/Mechanical/Rotational Elements/Mechanical Rotational Reference
  Saturation : Saturate  UpperLimit=1  LowerLimit=0
  Scope : Scope
      settings: ActiveDisplayYMinimum=-1.25  ActiveDisplayYMaximum=1.25
  Simulink-PS Converter : nesl_utility/Simulink-PS Converter  PhysicalDomain=network_engine_domain  SubClassName=ps_input  LeftPortType=input  RightPortType=output  PseudoPeriodic=off  Frequencies=[]  NoiseDistribution=none  NoiseParameters=[]  Unit=1  AffineConversion=off  FilteringAndDerivatives=zero  SimscapeFilterOrder=1  InputFilterTimeConstant=0.001  UdotUserProvided=1
  scale by base_torque : Gain  Gain=genRating*1000/(2*pi*frequency)
  R : PMIOPort  Side=Right
  C : PMIOPort  Port=2  Side=Right
  wires:
  Saturation/1 -> scale by base_torque/1
  scale by base_torque/1 -> Simulink-PS Converter/1
  PRef/1 -> Scope/1, Saturation/1
  connections:
  Simulink-PS Converter/RConn1 -- Ideal Torque Source/RConn1
  Ideal Torque Source/RConn2 -- Mechanical Rotational Reference/LConn1 -- C/RConn1
  Ideal Torque Source/LConn1 -- R/RConn1

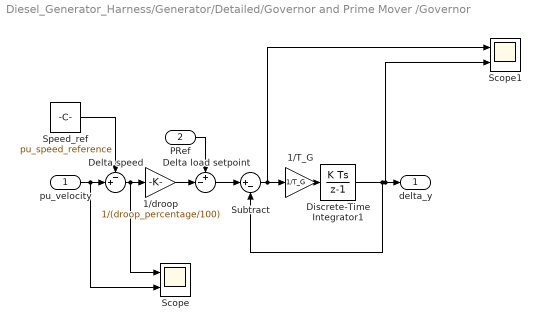
== system Diesel_Generator_Harness/Generator/Detailed/Governor and Prime Mover /Governor ==
  pu_velocity : Inport
  PRef : Inport  Port=2
  1/T_G : Gain  Gain=1/T_G
  1/droop : Gain  Gain=1/(droop_percentage/100)
  Delta load setpoint : Sum  Inputs=+-|
  Delta speed : Sum  Inputs=-+|
  Discrete-Time Integrator1 : DiscreteIntegrator  InitialCondition=pu_torque0  SampleTime=-1  ICPrevOutput=DiscIntNeverNeededParam  ICPrevScaledInput=DiscIntNeverNeededParam
  Scope : Scope  NumInputPorts=2
  Scope1 : Scope  NumInputPorts=2
  Speed_ref : Constant  Value=pu_speed_reference
  Subtract : Sum  Inputs=|+-
  delta_y : Outport  VectorParamsAs1DForOutWhenUnconnected=off
  wires:
  PRef/1 -> Delta load setpoint/1
  Discrete-Time Integrator1/1 -> Subtract/2, delta_y/1, Scope1/2
  1/T_G/1 -> Discrete-Time Integrator1/1
  Subtract/1 -> 1/T_G/1, Scope1/1
  Delta load setpoint/1 -> Subtract/1
  1/droop/1 -> Delta load setpoint/2
  pu_velocity/1 -> Delta speed/2, Scope/2
  Delta speed/1 -> 1/droop/1, Scope/1
  Speed_ref/1 -> Delta speed/1

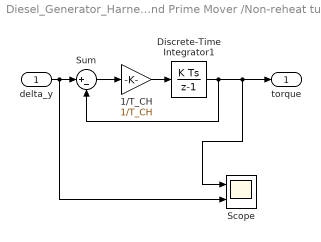
== system Diesel_Generator_Harness/Generator/Detailed/Governor and Prime Mover /Non-reheat turbine ==
  delta_y : Inport
  1/T_CH : Gain  Gain=1/T_CH
  Discrete-Time Integrator1 : DiscreteIntegrator  InitialCondition=pu_torque0  SampleTime=-1  ICPrevOutput=DiscIntNeverNeededParam  ICPrevScaledInput=DiscIntNeverNeededParam
  Scope : Scope  NumInputPorts=2
  Sum : Sum  Inputs=|+-
  torque : Outport  VectorParamsAs1DForOutWhenUnconnected=off
  wires:
  Discrete-Time Integrator1/1 -> torque/1, Scope/1, Sum/2
  1/T_CH/1 -> Discrete-Time Integrator1/1
  Sum/1 -> 1/T_CH/1
  delta_y/1 -> Sum/1, Scope/2
